simulink library "Lib_Rev2_Dvcu_IO"  (R2019b)
settings: Solver=ode45  StartTime=0.0  StopTime=10.0  RelTol=1e-3  EnableMultiTasking=on
settings Model: Creator=kmansour  LastModifiedBy=depl_
settings DataIOCC: LimitDataPoints=on  SaveFormat=Array  ReturnWorkspaceOutputs=off
settings OptimizationCC: LifeSpan=inf
settings DebuggingCC: AllowSymbolicDim=off  SFUnexpectedBacktrackingDiag=warning  SFNoUnconditionalDefaultTransitionDiag=warning  SFExecutionAtInitializationDiag=none  ArithmeticOperatorsInVariantConditions=warning
settings HardwareCC: ProdBitPerPointer=32  ProdBitPerSizeT=32  ProdBitPerPtrDiffT=32  ProdLargestAtomicFloat=None  ProdIntDivRoundTo=Undefined  ProdEndianess=Unspecified  ProdWordSize=32  ProdHWDeviceType=32-bit Generic
settings ModelReferenceCC: PropagateSignalLabelsOutOfModel=off
settings SFSimCC: SimUseLocalCustomCode=off  CustomCodeUndefinedFunction=UseInterfaceOnly
settings RTWCC: RTWUseLocalCustomCode=off
settings CodeAppCC: StateflowObjectComments=on
settings GRTTargetCC: TargetLangStandard=C89/C90 (ANSI)  GeneratePreprocessorConditionals=Disable all
settings ConfigComp: CovMetricSettings=dw  CovHtmlReporting=on  CovSaveCumulativeToWorkspaceVar=on  CovSaveSingleToWorkspaceVar=on  CovExternalEMLEnable=off

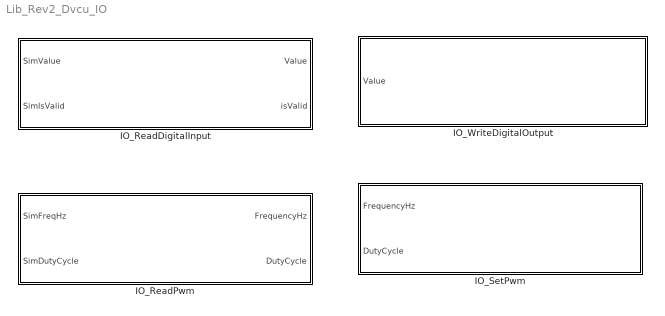
== system Lib_Rev2_Dvcu_IO ==
  IO_ReadDigitalInput : Subsystem  TreatAsAtomicUnit=on  mask{PARAM_ID=ECU_DIN_AUX_61_H_DI}
      mask prompts: PARAM_ID "Choose a Signal"
      mask TypeOptions PARAM_ID: ECU_DIN_AUX_61_H_DI | ECU_DIN_AUX_51_H_DI | ECU_DIN_AUX_22_H_DI | ECU_DIN_AUX_34_L_DI | ECU_DIN_AUX_27_H_DI | ECU_DIN_AUX_42_H_DI | ECU_DIN_AUX_21_H_DI | ECU_DIN_AUX_31_H_DI | ECU_DIN_AUX_23_H_DI | ECU_DIN_AUX_41_H_DI | ECU_DIN_AUX_37_H_DI | ECU_DIN_AUX_25_L_DI | ECU_DIN_AUX_26_L_DI | ECU_DIN_AUX_35_L_DI | ECU_DIN_AUX_33_H_DI | ECU_DIN_AUX_36_L_DI | ECU_DIN_AUX_24_H_DI | ECU_DIN_AUX_28_L_DI | ECU_DIN_AUX_38_L_DI
      mask Display:
      | image(imread('devcu_final.png'),'top-left');
      | color('black');
      | port_label('input', 1, 'SimValue');
      | port_label('input', 2, 'SimIsValid');
      | port_label('output', 1, 'Value');
      | port_label('output', 2, 'isValid');
      | 
      | strCell =get_param(gcb, 'MaskValues');
      | strCell = strtrim(strCell);
      | str = strCell{1};
      | str = strrep(str, '_', '\_');
      | disp(str, 'texmode', 'on');
  IO_ReadPwm : Subsystem  TreatAsAtomicUnit=on  mask{PARAM_ID=ECU_PIN_NONAME_PIN_P13}
      mask prompts: PARAM_ID "Choose a Signal"
      mask TypeOptions PARAM_ID: ECU_PIN_NONAME_PIN_P13 | ECU_PIN_NONAME_PIN_P14 | ECU_PIN_NONAME_PIN_P62
      mask Display:
      | image(imread('devcu_final.png'),'top-left');
      | color('black');
      | port_label('input', 1, 'SimFrequency(Hz)');
      | port_label('input', 2, 'SimDutyCycle(%)');
      | port_label('output', 1, 'Frequency(Hz)');
      | port_label('output', 2, 'DutyCycle(%)');
      | 
      | strCell =get_param(gcb, 'MaskValues');
      | strCell = strtrim(strCell);
      | str = strCell{1};
      | str = strrep(str, '_', '\_');
      | disp(str, 'texmode', 'on');
  IO_SetPwm : Subsystem  TreatAsAtomicUnit=on  mask{PARAM_ID=ECU_POUT_PWM_POUT_P16}
      mask prompts: PARAM_ID "Choose a Signal"
      mask TypeOptions PARAM_ID: ECU_POUT_PWM_POUT_P16 | ECU_POUT_PWM_POUT_P7 | ECU_POUT_PWM_POUT_P12 | ECU_POUT_PWM_POUT_P11 | ECU_POUT_PWM_POUT_H | ECU_POUT_PWM_POUT_P17
      mask Display:
      | image(imread('devcu_final.png'),'top-right');
      | color('black');
      | port_label('input', 1, 'Frequency(Hz)');
      | port_label('input', 2, 'DutyCycle(%)');
      | 
      | strCell =get_param(gcb, 'MaskValues');
      | strCell = strtrim(strCell);
      | str = strCell{1};
      | str = strrep(str, '_', '\_');
      | disp(str, 'texmode', 'on');
  IO_WriteDigitalOutput : Subsystem  TreatAsAtomicUnit=on  mask{PARAM_ID=ECU_DOUT_NONAME_PIN_P15}
      mask prompts: PARAM_ID "Choose an Output"
      mask TypeOptions PARAM_ID: ECU_DOUT_NONAME_PIN_P15 | ECU_DOUT_NONAME_PIN_P16 | ECU_DOUT_NONAME_PIN_P20 | ECU_DOUT_NONAME_PIN_P21 | ECU_DOUT_NONAME_PIN_P22 | ECU_DOUT_NONAME_PIN_P24 | ECU_DOUT_NONAME_PIN_P33 | ECU_DOUT_NONAME_PIN_P34 | ECU_DOUT_NONAME_PIN_P40 | ECU_DOUT_NONAME_PIN_P42 | ECU_DOUT_NONAME_PIN_P43 | ECU_DOUT_NONAME_PIN_P90 | ECU_DOUT_NONAME_PIN_P91 | ECU_DOUT_NONAME_PIN_P92 | ECU_DOUT_NONAME_PIN_P93 | ECU_DOUT_NONAME_PIN_P94
      mask Display:
      | image(imread('devcu_final.png'),'top-right');
      | color('black');
      | port_label('input', 1, 'Value');
      | 
      | strCell =get_param(gcb, 'MaskValues');
      | strCell = strtrim(strCell);
      | str = strCell{1};
      | str = strrep(str, '_', '\_');
      | disp(str, 'texmode', 'on');

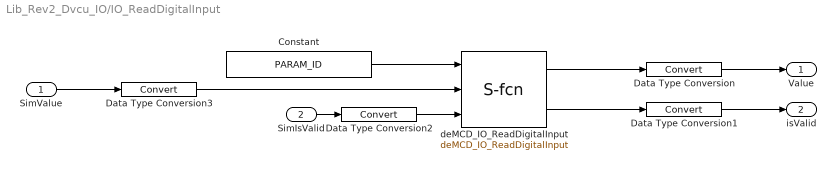
== system Lib_Rev2_Dvcu_IO/IO_ReadDigitalInput ==
  SimValue : Inport
  SimIsValid : Inport  Port=2
  Constant : Constant  Value=PARAM_ID
  Data Type Conversion{,1..3} (4 alike) : DataTypeConversion
  deMCD_IO_ReadDigitalInput : S-Function  FunctionName=deMCD_IO_ReadDigitalInput  SFunctionDeploymentMode=off  EnableBusSupport=off
      mask Display:
      | image(imread('logo_deMCD_white_background.png'),'center');
      | color('black');
      | port_label('input', 1, 'ID');
      | port_label('input', 2, 'SimValue');
      | port_label('input', 3, 'SimIsValid');
      | port_label('output', 1, 'Value');
      | port_label('output', 2, 'isReady');
  Value : Outport
  isValid : Outport  Port=2
  wires:
  deMCD_IO_ReadDigitalInput/1 -> Data Type Conversion/1
  Data Type Conversion/1 -> Value/1
  Constant/1 -> deMCD_IO_ReadDigitalInput/1
  deMCD_IO_ReadDigitalInput/2 -> Data Type Conversion1/1
  Data Type Conversion1/1 -> isValid/1
  SimIsValid/1 -> Data Type Conversion2/1
  Data Type Conversion3/1 -> deMCD_IO_ReadDigitalInput/2
  SimValue/1 -> Data Type Conversion3/1
  Data Type Conversion2/1 -> deMCD_IO_ReadDigitalInput/3

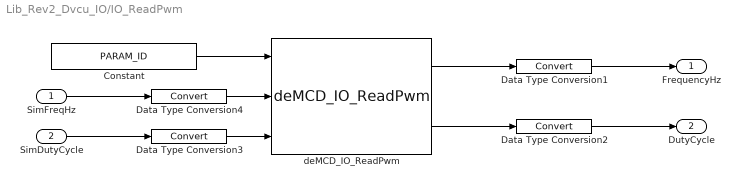
== system Lib_Rev2_Dvcu_IO/IO_ReadPwm ==
  SimFreqHz : Inport
  SimDutyCycle : Inport  Port=2
  Constant : Constant  Value=PARAM_ID
  Data Type Conversion{1..4} (4 alike) : DataTypeConversion
  deMCD_IO_ReadPwm : S-Function  FunctionName=deMCD_IO_ReadPwm  SFunctionDeploymentMode=off  EnableBusSupport=off
      mask Display:
      | image(imread('logo_deMCD_white_background.png'),'center');
      | color('black');
      | port_label('input', 1, 'ID');
      | port_label('input', 2, 'SimFrequency(Hz)');
      | port_label('input', 3, 'SimDutyCycle(%)');
      | port_label('output', 1, 'Frequency(Hz)');
      | port_label('output', 2, 'DutyCycle(%)')
  FrequencyHz : Outport
  DutyCycle : Outport  Port=2
  wires:
  Constant/1 -> deMCD_IO_ReadPwm/1
  deMCD_IO_ReadPwm/1 -> Data Type Conversion1/1
  deMCD_IO_ReadPwm/2 -> Data Type Conversion2/1
  Data Type Conversion1/1 -> FrequencyHz/1
  Data Type Conversion2/1 -> DutyCycle/1
  SimDutyCycle/1 -> Data Type Conversion3/1
  Data Type Conversion4/1 -> deMCD_IO_ReadPwm/2
  SimFreqHz/1 -> Data Type Conversion4/1
  Data Type Conversion3/1 -> deMCD_IO_ReadPwm/3

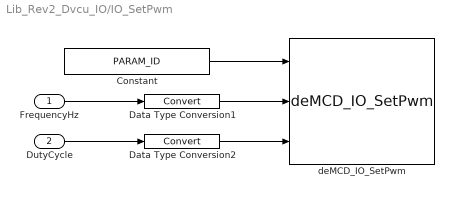
== system Lib_Rev2_Dvcu_IO/IO_SetPwm ==
  FrequencyHz : Inport
  DutyCycle : Inport  Port=2
  Constant : Constant  Value=PARAM_ID
  Data Type Conversion1 : DataTypeConversion
  Data Type Conversion2 : DataTypeConversion
  deMCD_IO_SetPwm : S-Function  FunctionName=deMCD_IO_SetPwm  SFunctionDeploymentMode=off  EnableBusSupport=off
      mask Display:
      | image(imread('logo_deMCD_white_background.png'),'center');
      | color('black');
      | port_label('input', 1, 'ID');
      | port_label('input', 2, 'Frequency(Hz)');
      | port_label('input', 3, 'DutyCycle(%)')
  wires:
  Constant/1 -> deMCD_IO_SetPwm/1
  DutyCycle/1 -> Data Type Conversion2/1
  FrequencyHz/1 -> Data Type Conversion1/1
  Data Type Conversion1/1 -> deMCD_IO_SetPwm/2
  Data Type Conversion2/1 -> deMCD_IO_SetPwm/3

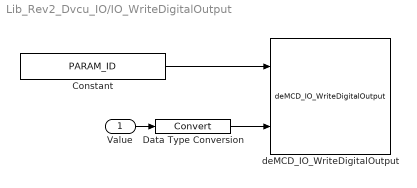
== system Lib_Rev2_Dvcu_IO/IO_WriteDigitalOutput ==
  Value : Inport
  Constant : Constant  Value=PARAM_ID
  Data Type Conversion : DataTypeConversion
  deMCD_IO_WriteDigitalOutput : S-Function  FunctionName=deMCD_IO_WriteDigitalOutput  SFunctionDeploymentMode=off  EnableBusSupport=off
      mask Display:
      | image(imread('logo_deMCD_white_background.png'),'center');
      | color('black');
      | port_label('input', 1, 'ID');
      | port_label('input', 2, 'Value');
  wires:
  Data Type Conversion/1 -> deMCD_IO_WriteDigitalOutput/2
  Constant/1 -> deMCD_IO_WriteDigitalOutput/1
  Value/1 -> Data Type Conversion/1
